simulink model "chap9_2"  (Simulink 3.00)
settings: Solver=ode45  StartTime=0.0  StopTime=20  RelTol=1e-3
values from neighbouring files (symbols this model uses):
  af = 0.02    [chap9_2i.m]
  J = 2    [Chap9_5i.m]    (also in chap9_1eq.m = 1; chap9_2i.m = 1; chap9_3.m = 0.6; chap9_4plant.m = 0.6)
  rou0 = 260    [chap9_2i.m]
  rou1 = 2.5    [chap9_2i.m]

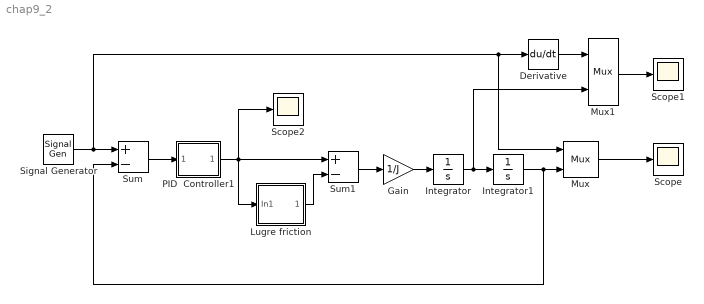
== system chap9_2 ==
  Derivative : Derivative
  Gain : Gain  Gain=1/J  SaturateOnIntegerOverflow=on
  Integrator : Integrator  ExternalReset=none  InitialConditionSource=internal  InitialCondition=0  LimitOutput=off  UpperSaturationLimit=inf  LowerSaturationLimit=-inf  ShowSaturationPort=off  ShowStatePort=off  AbsoluteTolerance=auto
  Integrator1 : Integrator  ExternalReset=none  InitialConditionSource=internal  InitialCondition=0  LimitOutput=off  UpperSaturationLimit=inf  LowerSaturationLimit=-inf  ShowSaturationPort=off  ShowStatePort=off  AbsoluteTolerance=auto
  Lugre friction : Subsystem
  Mux : Mux  Inputs=2
      settings: DisplayOption=none
  Mux1 : Mux  Inputs=2
      settings: DisplayOption=none
  PID  Controller1 : Subsystem  mask(PID Controller){@1=20, @2=0, @3=5}
      mask prompts: @1 "Proportional:"; @2 "Integral"; @3 "Derivative:"
      mask help:
      | Enter expressions for proportional, integral, and derivative terms.
      | P+I/s+Ds
      mask init:
      | P=@1; I=@2; D=@3;
      mask Help: This block implements a PID controller where parameters are entered for the Proportional, Integral and Derivative terms. Unmask this block to see how it works. The derivative term is implemented using a true derivative block.
      mask Display: disp('PID')
  Scope : Scope
      settings: TimeRange=1  YMin=-200  YMax=0  SaveToWorkspace=off  SaveName=ScopeData
  Scope1 : Scope
      settings: TimeRange=10  YMin=-1  YMax=1  SaveToWorkspace=off  SaveName=ScopeData
  Scope2 : Scope
      settings: TimeRange=1  YMin=-200  YMax=0  SaveToWorkspace=off  SaveName=ScopeData
  Signal Generator : SignalGenerator  WaveForm=sine  Amplitude=0.1  Frequency=0.10  Units=Hertz
  Sum : Sum  Inputs=+-  SaturateOnIntegerOverflow=on
  Sum1 : Sum  Inputs=+-  SaturateOnIntegerOverflow=on
  wires:
  Mux/1 -> Scope/1
  Integrator1/1 -> Mux/2, Sum/2
  Integrator/1 -> Integrator1/1, Mux1/2
  Lugre friction/1(Out1) -> Sum1/2
  Sum/1 -> PID  Controller1/1(In_1)
  PID  Controller1/1(Out_1) -> Lugre friction/1(In1), Sum1/1, Scope2/1
  Signal Generator/1 -> Sum/1, Mux/1, Derivative/1
  Gain/1 -> Integrator/1
  Sum1/1 -> Gain/1
  Mux1/1 -> Scope1/1
  Derivative/1 -> Mux1/1

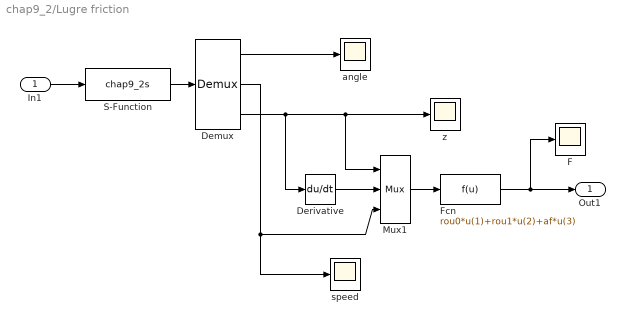
== system chap9_2/Lugre friction ==
  In1 : Inport  Port=1  PortWidth=-1  SampleTime=-1  DataType=auto
      settings: SignalType=auto
  Demux : Demux  Outputs=3
  Derivative : Derivative
  F : Scope
      settings: TimeRange=10  YMin=-1  YMax=1  SaveToWorkspace=off  SaveName=ScopeData
  Fcn : Fcn  Expr=rou0*u(1)+rou1*u(2)+af*u(3)
  Mux1 : Mux  Inputs=3
      settings: DisplayOption=none
  S-Function : S-Function  FunctionName=chap9_2s  PortCounts=[]  SFunctionModules=''
  angle : Scope
      settings: TimeRange=10  YMin=-1  YMax=1  SaveToWorkspace=off  SaveName=ScopeData
  speed : Scope
      settings: TimeRange=10  YMin=-1  YMax=1  SaveToWorkspace=off  SaveName=ScopeData
  z : Scope
      settings: TimeRange=10  YMin=-1  YMax=1  SaveToWorkspace=off  SaveName=ScopeData
  Out1 : Outport  Port=1
  wires:
  S-Function/1 -> Demux/1
  Demux/3 -> Derivative/1, Mux1/1, z/1
  Derivative/1 -> Mux1/2
  Mux1/1 -> Fcn/1
  Demux/1 -> angle/1
  Demux/2 -> Mux1/3, speed/1
  Fcn/1 -> Out1/1, F/1
  In1/1 -> S-Function/1

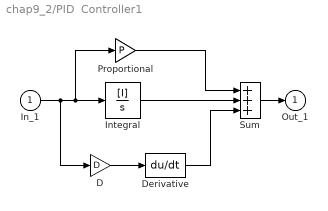
== system chap9_2/PID  Controller1 ==
  In_1 : Inport  Port=1  PortWidth=-1  SampleTime=-1  DataType=auto
      settings: SignalType=auto
  D : Gain  Gain=D  SaturateOnIntegerOverflow=on
  Derivative : Derivative
  Integral : TransferFcn  Numerator=[I]  Denominator=[1 0]
  Proportional : Gain  Gain=P  SaturateOnIntegerOverflow=on
  Sum : Sum  Inputs=+++  SaturateOnIntegerOverflow=on
  Out_1 : Outport  Port=1  InitialOutput=0
  wires:
  D/1 -> Derivative/1
  Sum/1 -> Out_1/1
  In_1/1 -> D/1, Proportional/1, Integral/1
  Derivative/1 -> Sum/3
  Integral/1 -> Sum/2
  Proportional/1 -> Sum/1
